simulink model "EE405L_Lab2_E1"  (R2021b)
settings: Solver=VariableStepAuto  StartTime=0.0  StopTime=10.0  RelTol=1e-3
undefined symbols (not defined in the file or in its folder): B, K, M
settings Model: Creator=Kevin  LastModifiedBy=Kevin

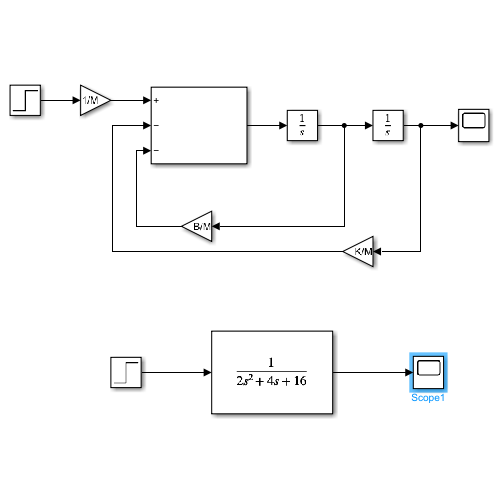
[thumbnail: Simulink's stored preview of the top-level diagram]
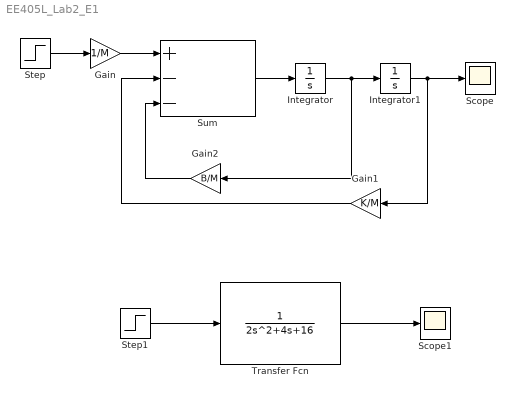
== system EE405L_Lab2_E1 ==
  Gain : Gain  Gain=1/M
  Gain1 : Gain  Gain=K/M
  Gain2 : Gain  Gain=B/M
  Integrator : Integrator
  Integrator1 : Integrator
  Scope : Scope
  Scope1 : Scope
  Step : Step  SampleTime=0
  Step1 : Step  SampleTime=0
  Sum : Sum  Inputs=+--
  Transfer Fcn : TransferFcn  Denominator=[2 4 16]
  wires:
  Step/1 -> Gain/1
  Gain/1 -> Sum/1
  Sum/1 -> Integrator/1
  Integrator/1 -> Gain2/1, Integrator1/1
  Integrator1/1 -> Gain1/1, Scope/1
  Gain2/1 -> Sum/3
  Gain1/1 -> Sum/2
  Step1/1 -> Transfer Fcn/1
  Transfer Fcn/1 -> Scope1/1
